simulink model "rider_model_ver3"  (R2018b)
settings: Solver=ode4  StartTime=0.0  StopTime=32.1780000000000  FixedStep=1e-3  MaxStep=1e-3  MinStep=1e-5  RelTol=1e-3
values from neighbouring files (symbols this model uses):
  K2 = whipple.K2    [delftbike.m]    (also in delftbikeHeading2.m = K2 .* a; getbicycleEOM.m = K2 .* a)
undefined symbols (not defined in the file or in its folder): K1
settings Model: Creator=chris  LastModifiedBy=chris

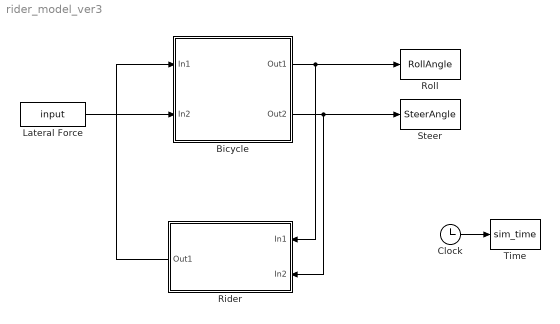
== system rider_model_ver3 ==
  Bicycle : Subsystem
  Clock : Clock
  Lateral Force : FromWorkspace  VariableName=input  SampleTime=0
  Rider : Subsystem
  Roll : ToWorkspace  VariableName=RollAngle  SampleTime=-1
  Steer : ToWorkspace  VariableName=SteerAngle  SampleTime=-1
  Time : ToWorkspace  VariableName=sim_time  SampleTime=-1
  wires:
  Bicycle/2(Out2) -> Steer/1, Rider/2(In2)
  Rider/1(Out1) -> Bicycle/1(In1)
  Lateral Force/1 -> Bicycle/2(In2)
  Bicycle/1(Out1) -> Roll/1, Rider/1(In1)
  Clock/1 -> Time/1

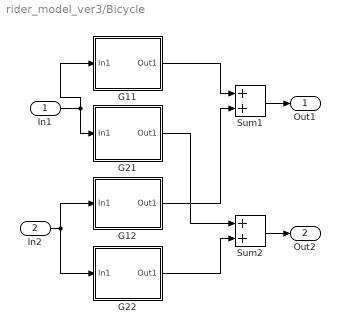
== system rider_model_ver3/Bicycle ==
  In1 : Inport
  In2 : Inport  Port=2
  G11 : Subsystem
  G12 : Subsystem
  G21 : Subsystem
  G22 : Subsystem
  Sum1 : Sum  SaturateOnIntegerOverflow=on  InputSameDT=on  OutDataTypeStr=Inherit: Same as first input
  Sum2 : Sum  SaturateOnIntegerOverflow=on  InputSameDT=on  OutDataTypeStr=Inherit: Same as first input
  Out1 : Outport  InitialOutput=0
  Out2 : Outport  Port=2  InitialOutput=0
  wires:
  In1/1 -> G11/1(In1), G21/1(In1)
  G21/1(Out1) -> Sum2/1
  G12/1(Out1) -> Sum1/2
  G11/1(Out1) -> Sum1/1
  G22/1(Out1) -> Sum2/2
  In2/1 -> G12/1(In1), G22/1(In1)
  Sum1/1 -> Out1/1
  Sum2/1 -> Out2/1

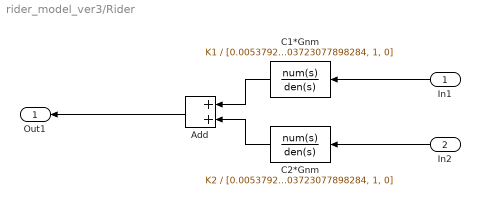
== system rider_model_ver3/Rider ==
  In1 : Inport
  In2 : Inport  Port=2
  Add : Sum
  C1*Gnm : TransferFcn  Numerator=K1  Denominator="[0.00537923844434676\t,0.103723077898284,\t1, 0]"
  C2*Gnm : TransferFcn  Numerator=K2  Denominator="[0.00537923844434676\t,0.103723077898284,\t1, 0]"
  Out1 : Outport
  wires:
  Add/1 -> Out1/1
  In1/1 -> C1*Gnm/1
  In2/1 -> C2*Gnm/1
  C2*Gnm/1 -> Add/2
  C1*Gnm/1 -> Add/1

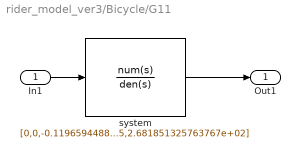
== system rider_model_ver3/Bicycle/G11 ==
  In1 : Inport
  system : TransferFcn  Numerator=[0,0,-0.119659448859188,-6.366433554305944,-46.227590882295810]  Denominator=[1,11.155335783994320,-13.554033257307804,12.022586791665745,2.681851325763767e+02]
  Out1 : Outport  InitialOutput=0
  wires:
  In1/1 -> system/1
  system/1 -> Out1/1

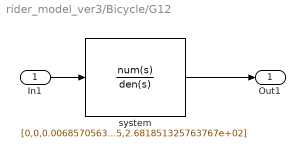
== system rider_model_ver3/Bicycle/G12 ==
  In1 : Inport
  system : TransferFcn  Numerator=[0,0,0.006857056322092,0.081095421172526,-0.060229564608997]  Denominator=[1,11.155335783994320,-13.554033257307804,12.022586791665745,2.681851325763767e+02]
  Out1 : Outport  InitialOutput=0
  wires:
  In1/1 -> system/1
  system/1 -> Out1/1

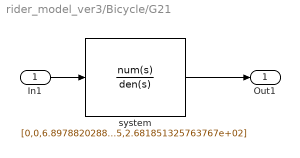
== system rider_model_ver3/Bicycle/G21 ==
  In1 : Inport
  system : TransferFcn  Numerator=[0,0,6.897882028828916,0,-56.373199257664180]  Denominator=[1,11.155335783994320,-13.554033257307804,12.022586791665745,2.681851325763767e+02]
  Out1 : Outport  InitialOutput=0
  wires:
  In1/1 -> system/1
  system/1 -> Out1/1

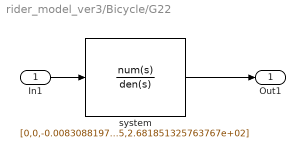
== system rider_model_ver3/Bicycle/G22 ==
  In1 : Inport
  system : TransferFcn  Numerator=[0,0,-0.008308819701902,0.084055364204546,0.195185649792306]  Denominator=[1,11.155335783994320,-13.554033257307804,12.022586791665745,2.681851325763767e+02]
  Out1 : Outport  InitialOutput=0
  wires:
  In1/1 -> system/1
  system/1 -> Out1/1
